simulink model "debug_positionControl"  (Simulink 10.1)
settings: Solver=FixedStepDiscrete  StartTime=0.0  StopTime=inf  FixedStep=0.01  RelTol=1e-3
libraries: WBToolboxLibrary x15
settings Model: Creator=sdafarra  LastModifiedBy=sdafarra
settings DataIOCC: SaveFormat=Dataset  ReturnWorkspaceOutputs=on
settings OptimizationCC: LifeSpan=auto
settings DebuggingCC: UnderspecifiedInitializationDetection=Simplified  MergeDetectMultiDrivingBlocksExec=error  SFUnexpectedBacktrackingDiag=error  SFNoUnconditionalDefaultTransitionDiag=error  SFExecutionAtInitializationDiag=warning  ArithmeticOperatorsInVariantConditions=error
settings HardwareCC: ProdBitPerPointer=64  ProdBitPerSizeT=64  ProdBitPerPtrDiffT=64  ProdLargestAtomicFloat=Float  ProdIntDivRoundTo=Zero  ProdEndianess=LittleEndian  ProdWordSize=64  ProdHWDeviceType=Intel->x86-64 (Windows64)
settings ModelReferenceCC: PropagateSignalLabelsOutOfModel=on
settings SFSimCC: SimUseLocalCustomCode=on  CustomCodeUndefinedFunction=FilterOut
settings RTWCC: RTWUseLocalCustomCode=on
settings CodeAppCC: StateflowObjectComments=off
settings GRTTargetCC: TargetLangStandard=C99 (ISO)  CombineOutputUpdateFcns=on  GRTInterface=off
settings ConfigComp: CovMetricSettings=dwe  CovHtmlReporting=off  CovSaveCumulativeToWorkspaceVar=off  CovSaveSingleToWorkspaceVar=off  CovExternalEMLEnable=on

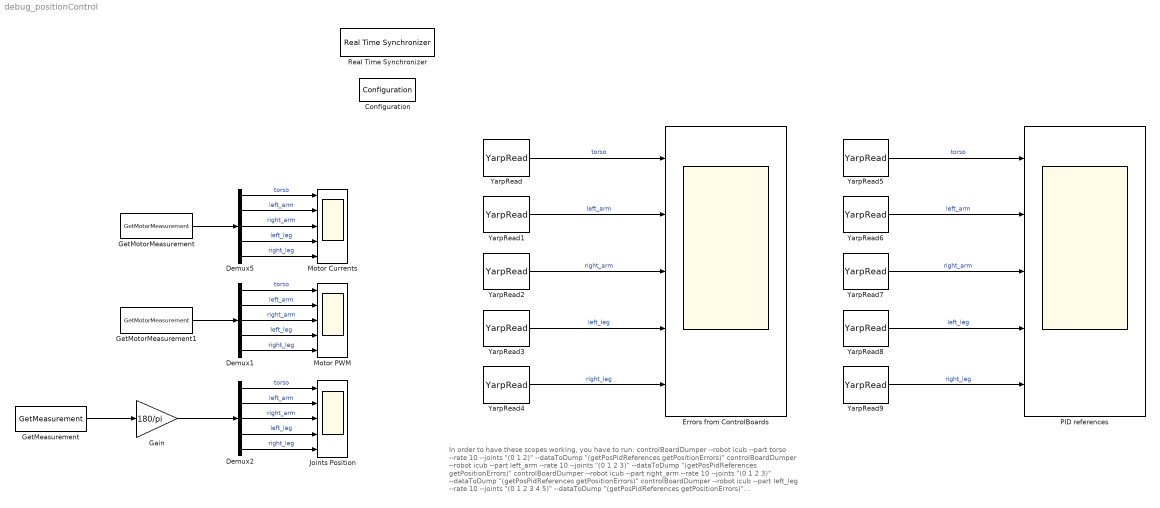
== system debug_positionControl ==
  note: In order to have these scopes working, you have to run:
      | controlBoardDumper --robot icub --part torso --rate 10 --joints "(0 1 2)" --dataToDump "(getPosPidReferences getPositionErrors)"
      | controlBoardDumper --robot icub --part left_arm --rate 10 --joints "(0 1 2 3)" --dataToDump "(getPosPidReferences getPositionErrors)"
      | controlBoardDumper --robot icub --part right_arm --rate 10 --joints "(0 1 2 3)" --dataToDump "(getPosPidReferences getPositionErrors)"
      | controlBoardDumper --robot icub --part left_leg --rate 10 --joints "(0 1 2 3 4 5)" --dataToDump "(getPosPidReferences getPositionErrors)"
      | controlBoardDumper --robot icub --part right_leg --rate 10 --joints "(0 1 2 3 4 5)" --dataToDump "(getPosPidReferences getPositionErrors)"
      |
      | On Linux environments, you can simply run the following, unique, command on a terminal:
      |
      | (controlBoardDumper --robot icub --part torso --rate 10 --joints "(0 1 2)" --dataToDump "(getPosPidReferences getPositionErrors)" & controlBoardDumper --robot icub --part left_arm --rate 10 --joints "(0 1 2 3)" --dataToDump "(getPosPidReferences getPositionErrors)" & controlBoardDumper --robot icub --part right_arm --rate 10 --joints "(0 1 2 3)" --dataToDump "(getPosPidReferences getPositionErrors)" & controlBoardDumper --robot icub --part left_leg --rate 10 --joints "(0 1 2 3 4 5)" --dataToDump "(getPosPidReferences getPositionErrors)" & controlBoardDumper --robot icub --part right_leg --rate 10 --joints "(0 1 2 3 4 5)" --dataToDump "(getPosPidReferences getPositionErrors)" & wait)
  Configuration : WBToolboxLibrary/Utilities/Configuration  ConfigSource=Mask  ConfigObject='WBTConfigRobot'  RobotName='icub'  UrdfFile='model.urdf'  ControlledJoints={'torso_pitch','torso_roll','torso_yaw','l_shoulder_pitch','l_shoulder_roll','l_shoulder_yaw','l_elbow','r_shoulder_pitch','r_shoulder_roll','r_shoulder_yaw','r_elbow','l_hip_pitch','l_hip_roll','l_hip_yaw','l_knee','l_ankle_pitch','l_ankle_roll', 'r_hip_pitch','r_hip_roll','r_hip_yaw','r_knee','r_ankle_pitch','r_ankle_roll'}  ControlBoardsNames={'torso','left_arm','right_arm','left_leg','right_leg'}  LocalName='WBT'  GravityVector=[0,0,-9.81]
      settings: SourceProductName=Whole Body Toolbox
  Demux1 : Demux  Outputs=[3,4,4,6,6]
  Demux2 : Demux  Outputs=[3,4,4,6,6]
  Demux5 : Demux  Outputs=[3,4,4,6,6]
  Errors from ControlBoards : Scope  NumInputPorts=5
  Gain : Gain  Gain=180/pi
  GetMeasurement : WBToolboxLibrary/States/GetMeasurement  measuredType=Joints Position
      settings: SourceProductName=WholeBodyToolbox
  GetMotorMeasurement : WBToolboxLibrary/States/GetMotorMeasurement  measuredType=Motor Current
      settings: SourceProductName=WholeBodyToolbox
  GetMotorMeasurement1 : WBToolboxLibrary/States/GetMotorMeasurement  measuredType=Motor PWM
      settings: SourceProductName=WholeBodyToolbox
  Joints Position : Scope  NumInputPorts=5
  Motor Currents : Scope  NumInputPorts=5
  Motor PWM : Scope  NumInputPorts=5
  PID references : Scope  NumInputPorts=5
  Real Time Synchronizer : WBToolboxLibrary/Utilities/Real Time Synchronizer  period=0.01
      settings: SourceProductName=Whole Body Toolbox
  YarpRead : WBToolboxLibrary/Utilities/YarpRead  portName='/controlBoardDumper/torso/getPositionErrors'  signalSize=3  timeout=0.5  blocking=off  timestamp=off  autoconnect=on  errorOnConnection=on
      settings: SourceProductName=WholeBodyToolbox
  YarpRead1 : WBToolboxLibrary/Utilities/YarpRead  portName='/controlBoardDumper/left_arm/getPositionErrors'  signalSize=4  timeout=0.5  blocking=off  timestamp=off  autoconnect=on  errorOnConnection=on
      settings: SourceProductName=WholeBodyToolbox
  YarpRead2 : WBToolboxLibrary/Utilities/YarpRead  portName='/controlBoardDumper/right_arm/getPositionErrors'  signalSize=4  timeout=0.5  blocking=off  timestamp=off  autoconnect=on  errorOnConnection=on
      settings: SourceProductName=WholeBodyToolbox
  YarpRead3 : WBToolboxLibrary/Utilities/YarpRead  portName='/controlBoardDumper/left_leg/getPositionErrors'  signalSize=6  timeout=0.5  blocking=off  timestamp=off  autoconnect=on  errorOnConnection=on
      settings: SourceProductName=WholeBodyToolbox
  YarpRead4 : WBToolboxLibrary/Utilities/YarpRead  portName='/controlBoardDumper/right_leg/getPositionErrors'  signalSize=6  timeout=0.5  blocking=off  timestamp=off  autoconnect=on  errorOnConnection=on
      settings: SourceProductName=WholeBodyToolbox
  YarpRead5 : WBToolboxLibrary/Utilities/YarpRead  portName='/controlBoardDumper/torso/getPosPidReferences'  signalSize=3  timeout=0.5  blocking=off  timestamp=off  autoconnect=on  errorOnConnection=on
      settings: SourceProductName=WholeBodyToolbox
  YarpRead6 : WBToolboxLibrary/Utilities/YarpRead  portName='/controlBoardDumper/left_arm/getPosPidReferences'  signalSize=4  timeout=0.5  blocking=off  timestamp=off  autoconnect=on  errorOnConnection=on
      settings: SourceProductName=WholeBodyToolbox
  YarpRead7 : WBToolboxLibrary/Utilities/YarpRead  portName='/controlBoardDumper/right_arm/getPosPidReferences'  signalSize=4  timeout=0.5  blocking=off  timestamp=off  autoconnect=on  errorOnConnection=on
      settings: SourceProductName=WholeBodyToolbox
  YarpRead8 : WBToolboxLibrary/Utilities/YarpRead  portName='/controlBoardDumper/left_leg/getPosPidReferences'  signalSize=6  timeout=0.5  blocking=off  timestamp=off  autoconnect=on  errorOnConnection=on
      settings: SourceProductName=WholeBodyToolbox
  YarpRead9 : WBToolboxLibrary/Utilities/YarpRead  portName='/controlBoardDumper/right_leg/getPosPidReferences'  signalSize=6  timeout=0.5  blocking=off  timestamp=off  autoconnect=on  errorOnConnection=on
      settings: SourceProductName=WholeBodyToolbox
  wires:
  GetMotorMeasurement/1 -> Demux5/1
  GetMotorMeasurement1/1 -> Demux1/1
  YarpRead1/1 -> Errors from ControlBoards/2  "left_arm"
  YarpRead2/1 -> Errors from ControlBoards/3  "right_arm"
  YarpRead3/1 -> Errors from ControlBoards/4  "left_leg"
  YarpRead/1 -> Errors from ControlBoards/1  "torso"
  YarpRead4/1 -> Errors from ControlBoards/5  "right_leg"
  YarpRead8/1 -> PID references/4  "left_leg"
  YarpRead5/1 -> PID references/1  "torso"
  YarpRead7/1 -> PID references/3  "right_arm"
  YarpRead6/1 -> PID references/2  "left_arm"
  YarpRead9/1 -> PID references/5  "right_leg"
  Demux5/1 -> Motor Currents/1  "torso"
  Demux5/2 -> Motor Currents/2  "left_arm"
  Demux5/3 -> Motor Currents/3  "right_arm"
  Demux5/4 -> Motor Currents/4  "left_leg"
  Demux5/5 -> Motor Currents/5  "right_leg"
  Demux1/1 -> Motor PWM/1  "torso"
  Demux1/2 -> Motor PWM/2  "left_arm"
  Demux1/3 -> Motor PWM/3  "right_arm"
  Demux1/4 -> Motor PWM/4  "left_leg"
  Demux1/5 -> Motor PWM/5  "right_leg"
  Demux2/1 -> Joints Position/1  "torso"
  Demux2/2 -> Joints Position/2  "left_arm"
  Demux2/3 -> Joints Position/3  "right_arm"
  Demux2/4 -> Joints Position/4  "left_leg"
  Demux2/5 -> Joints Position/5  "right_leg"
  GetMeasurement/1 -> Gain/1
  Gain/1 -> Demux2/1
